simulink model "heli_state_observer"  (R2020a)
settings: Solver=ode4  StartTime=0.0  StopTime=inf  FixedStep=0.1  RelTol=1e-3
values from neighbouring files (symbols this model uses):
  A = ds.A    [initialize_system.m]
  B = ds.B    [initialize_system.m]
  C = ds.C    [initialize_system.m]
undefined symbols (not defined in the file or in its folder): L
settings Model: Creator=engen  LastModifiedBy=engen

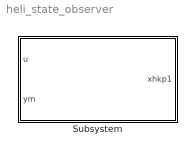
== system heli_state_observer ==
  Subsystem : Subsystem

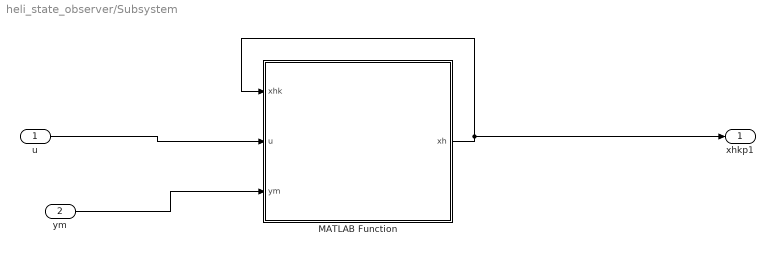
== system heli_state_observer/Subsystem ==
  u : Inport
  ym : Inport  Port=2
  MATLAB Function : MATLAB Function  TreatAsAtomicUnit=on
  xhkp1 : Outport
  wires:
  MATLAB Function/1(xh) -> MATLAB Function/1(xhk), xhkp1/1
  ym/1 -> MATLAB Function/3(ym)
  u/1 -> MATLAB Function/2(u)

== matlab function heli_state_observer/Subsystem/MATLAB Function ==
  data: xhk input; u input; xh output; ym input; A parameter; L parameter; B parameter; C parameter
function xh = fcn(xhk,u,ym,A, L, B, C)
xhkp1 = A*xhk+B*u+L*(ym-C*xhk);
xh = xhkp1;
